simulink model "Project2LateralDynamics"  (R2024a)
settings: Solver=VariableStepAuto  StartTime=0.0  StopTime=10.0  RelTol=1e-3
settings Model: Creator=Joseph  LastModifiedBy=Joseph
settings DataIOCC: ExternalInput=[t, u, obj]  LoadExternalInput=on

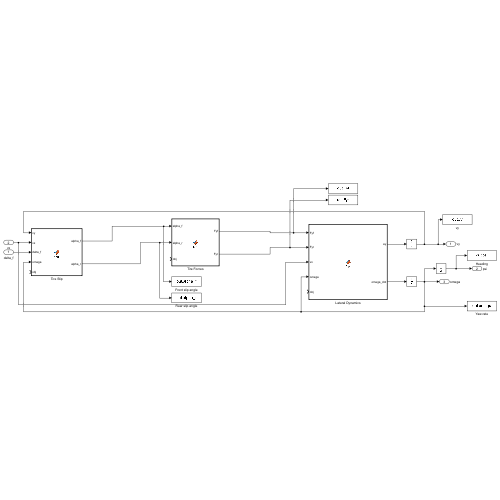
[thumbnail: Simulink's stored preview of the top-level diagram]
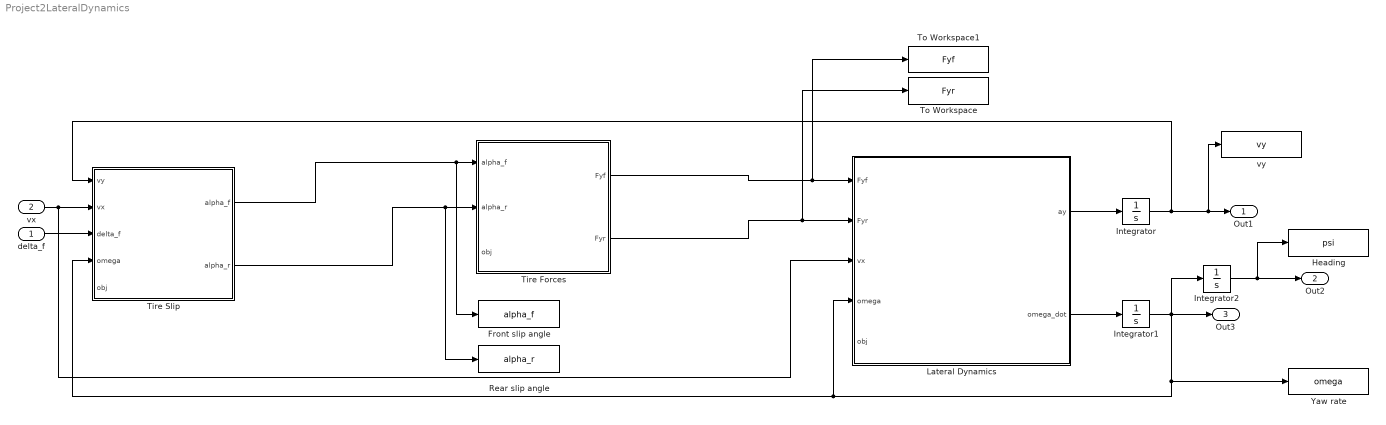
== system Project2LateralDynamics ==
  delta_f : Inport
  vx : Inport  Port=2
  Front slip angle : ToWorkspace  VariableName=alpha_f  SaveFormat=Timeseries  SampleTime=-1
  Heading : ToWorkspace  VariableName=psi  SaveFormat=Timeseries  SampleTime=-1
  Integrator : Integrator
  Integrator1 : Integrator
  Integrator2 : Integrator
  Lateral Dynamics : MATLAB Function  TreatAsAtomicUnit=on
  Rear slip angle : ToWorkspace  VariableName=alpha_r  SaveFormat=Timeseries  SampleTime=-1
  Tire Forces : MATLAB Function  TreatAsAtomicUnit=on
  Tire Slip : MATLAB Function  TreatAsAtomicUnit=on
  To Workspace : ToWorkspace  VariableName=Fyr  SaveFormat=Timeseries  SampleTime=-1
  To Workspace1 : ToWorkspace  VariableName=Fyf  SaveFormat=Timeseries  SampleTime=-1
  Yaw rate : ToWorkspace  VariableName=omega  SaveFormat=Timeseries  SampleTime=-1
  vy : ToWorkspace  VariableName=vy  SaveFormat=Timeseries  SampleTime=-1
  Out1 : Outport  SignalName=vy
  Out2 : Outport  Port=2  SignalName=psi
  Out3 : Outport  Port=3  SignalName=omega
  wires:
  Lateral Dynamics/1(ay) -> Integrator/1
  Integrator/1 -> vy/1, Out1/1, Tire Slip/1(vy)
  Tire Slip/1(alpha_f) -> Front slip angle/1, Tire Forces/1(alpha_f)
  Tire Slip/2(alpha_r) -> Rear slip angle/1, Tire Forces/2(alpha_r)
  Tire Forces/1(Fyf) -> To Workspace1/1, Lateral Dynamics/1(Fyf)
  Tire Forces/2(Fyr) -> To Workspace/1, Lateral Dynamics/2(Fyr)
  Lateral Dynamics/2(omega_dot) -> Integrator1/1
  Integrator1/1 -> Yaw rate/1, Tire Slip/4(omega), Lateral Dynamics/4(omega), Out3/1, Integrator2/1
  vx/1 -> Lateral Dynamics/3(vx), Tire Slip/2(vx)
  delta_f/1 -> Tire Slip/3(delta_f)
  Integrator2/1 -> Heading/1, Out2/1

== matlab function Project2LateralDynamics/Tire Forces ==
  data: alpha_f input; Fyf output; alpha_r input; Fyr output; obj input
function [Fyf, Fyr]= fcn(alpha_f, alpha_r, obj)

Fyf = min(obj.Fyfmax, obj.Calpha_f*alpha_f);
Fyr = min(obj.Fyrmax, obj.Calpha_r*alpha_r);
end

== matlab function Project2LateralDynamics/Tire Slip ==
  data: vy input; alpha_f output; vx input; delta_f input; omega input; alpha_r output; obj input
function [alpha_f, alpha_r]= fcn(vy, vx, delta_f, omega, obj)

if abs(vx) > obj.vx_threshold1
    alpha_f = delta_f - (vy + omega*obj.lf)/vx;
    alpha_r = -(vy - omega*obj.lr)/vx;
else
    alpha_f = 0;
    alpha_r = 0;
end
end

== matlab function Project2LateralDynamics/Lateral Dynamics ==
  data: Fyf input; ay output; Fyr input; vx input; omega input; omega_dot output; obj input
function [ay, omega_dot]= fcn(Fyf, Fyr, vx, omega, obj)

Fy = Fyf + Fyr;
ay = Fy/obj.Mass - omega*vx;
M = Fyf*obj.lf - Fyr*obj.lr;
omega_dot = M/obj.Inertia;
end
